simulink model "pmc_gpio_s32k11x"  (Simulink 9.0)
settings: Solver=FixedStepDiscrete  StartTime=0.0  StopTime=10.0  FixedStep=0.25  RelTol=1e-3
InitFcn:
  | mbd_s32k_consistency_checks(bdroot(gcs));
undefined symbols (not defined in the file): LQFP, thumb
libraries: mbd_s32k1xx_ec_toolbox x27, simulink x1
Description:
  | This model demonstrates the "Power Management" functionality by setting
  | the S32k144 controller in all power modes one at a time.
  | 
  | Validation: When the processor boots up, it enters the RUN power mode.  The SW3 switch
  | increments the sleep_state variable. It switches the power mode state according to the
  | sleep_state value. For every power mode, the RGB led lights up another colour:
  | RUN     - green
  | HSRUN - blue
  | STOP1 - yellow
  | STOP2 - magenta
  | VLPS   - red
  | To wake up the processor SW2 must be pressed.
  | 
  | Optional: In order to measure the current consumption of the processor you can desolder
  | the R117 resistor (on the S32K144EVB board) and attach an ammeter on the J15 jumper.
  | 
  | Warning: Do NOT program the board while the uC is running in the VLPR mode!
settings Model: Creator=NXP MBDT Team  LastModifiedBy=nxf35172
settings DataIOCC: ExternalInput=off  InitialState=off  SaveFormat=Dataset  SaveOutput=off  SignalLogging=off  SaveTime=off
settings OptimizationCC: DefaultParameterBehavior=Inlined  PassReuseOutputArgsAs=Individual arguments  LifeSpan=auto
settings DebuggingCC: UnderspecifiedInitializationDetection=Simplified  MergeDetectMultiDrivingBlocksExec=error  InheritedTsInSrcMsg=none  SingleTaskRateTransMsg=error  ParameterTunabilityLossMsg=error  UnconnectedInputMsg=error  UnconnectedOutputMsg=error  UnconnectedLineMsg=error  UnknownTsInhSupMsg=error  SFUnexpectedBacktrackingDiag=error  SFNoUnconditionalDefaultTransitionDiag=error
settings HardwareCC: ProdLargestAtomicInteger=Long  ProdLargestAtomicFloat=Double  ProdIntDivRoundTo=Zero  ProdEndianess=LittleEndian  ProdHWDeviceType=ARM Compatible->ARM Cortex
settings ModelReferenceCC: PropagateSignalLabelsOutOfModel=on
settings SFSimCC: MATLABDynamicMemAlloc=off
settings RTWCC: SystemTargetFile=mbd_s32k.tlc  MakeCommand=mbd_s32k_make_rtw COPY_MDLREF_INCLUDES=0  TemplateMakefile=mbd_s32k.tmf  Description=Model Based Design Toolbox S32K14x Code Generation Target  GenerateReport=on  RetainRTWFile=on  IncludeHyperlinkInReport=on  LaunchReport=on  GenerateTraceInfo=on  GenerateTraceReport=on  GenerateTraceReportSl=on  GenerateTraceReportSf=on  GenerateTraceReportEml=on
settings CodeAppCC: ForceParamTrailComments=on  IgnoreCustomStorageClasses=off  OperatorAnnotations=on  SimulinkDataObjDesc=on  SFDataObjDesc=on  InsertBlockDesc=on  StateflowObjectComments=off
settings STFCustomTargetCC: MultiwordLength=256  CombineOutputUpdateFcns=on  ERTCustomFileBanners=on  SupportContinuousTime=off  SupportNonInlinedSFcns=off  RemoveResetFunc=on  MATLABClassNameForMDSCustomization=Simulink.SoftwareTarget.ERTCustomization  GRTInterface=off  SystemTargetFile=mbd_s32k.tlc
settings ERTTargetCC: ParMdlRefBuildCompliant=off  CompOptLevelCompliant=off  ConcurrentExecutionCompliant=off  ModelStepFunctionPrototypeControlCompliant=off  CPPClassGenCompliant=off  UseToolchainInfoCompliant=off  InlinedParameterPlacement=NonHierarchical  ERTSrcFileBannerTemplate=mbd_ert_code_template.cgt  ERTHdrFileBannerTemplate=mbd_ert_code_template.cgt  ERTDataSrcFileTemplate=mbd_ert_code_template.cgt  ERTDataHdrFileTemplate=mbd_ert_code_template.cgt  ERTCustomFileTemplate=example_file_process.tlc
settings ConfigComp: CovMetricSettings=dwe  CovHtmlReporting=off  CovSaveCumulativeToWorkspaceVar=off  CovSaveSingleToWorkspaceVar=off  CovExternalEMLEnable=on

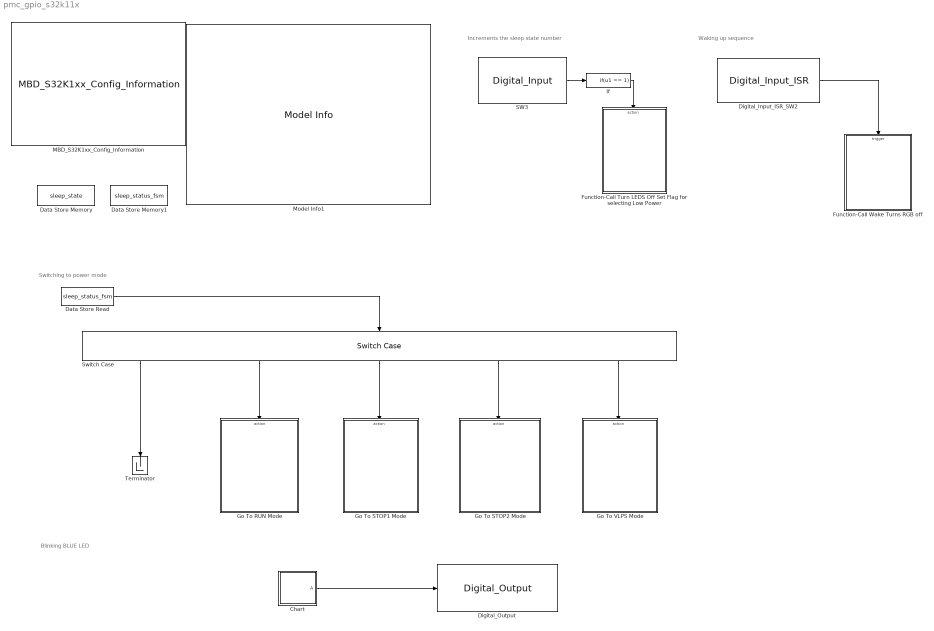
== system pmc_gpio_s32k11x ==
  note: Increments the sleep state number
  note: Waking up sequence
  note: Switching to power mode
  note: Blinking BLUE LED
  Chart : Stateflow chart  TreatAsAtomicUnit=on
  Data Store Memory : DataStoreMemory  DataStoreName=sleep_state  ReadBeforeWriteMsg=warning  WriteAfterWriteMsg=warning  WriteAfterReadMsg=warning  InitialValue=1  ShowAdditionalParam=off  OutDataTypeStr=uint8
  Data Store Memory1 : DataStoreMemory  DataStoreName=sleep_status_fsm  ReadBeforeWriteMsg=warning  WriteAfterWriteMsg=warning  WriteAfterReadMsg=warning  InitialValue=1  ShowAdditionalParam=off  OutDataTypeStr=uint8
  Data Store Read : DataStoreRead  DataStoreName=sleep_status_fsm
  Digital_Input_ISR_SW2 : mbd_s32k1xx_ec_toolbox/GPIO Blocks/Digital_Input_ISR  gpio_pin=PTD5: [PTD5 | Port D I/O]  irqc=on rising-edge  prio=0
  Digital_Output : mbd_s32k1xx_ec_toolbox/GPIO Blocks/Digital_Output  gpio_pin=PTE8: [PTE8 | Port E I/O]  init_val=Low  drive_strength=Low
  Function-Call Turn LEDS Off Set Flag for selecting Low Power : Subsystem  TreatAsAtomicUnit=on
  Function-Call Wake Turns RGB off : Subsystem  TreatAsAtomicUnit=on
  Go To RUN Mode : Subsystem  TreatAsAtomicUnit=on
  Go To STOP1 Mode : Subsystem  TreatAsAtomicUnit=on
  Go To STOP2 Mode : Subsystem  TreatAsAtomicUnit=on
  Go To VLPS Mode : Subsystem  TreatAsAtomicUnit=on
  If : If  IfExpression=u1 == 1  ShowElse=off
  MBD_S32K1xx_Config_Information : mbd_s32k1xx_ec_toolbox/MBD_S32K1xx_Config_Information  mbdt_ver=0  disp_str=|  config_params=[]  mcu_target_name=S32K116  mcu_target_package=48-LQFP  mcu_target_sram_size=17KB  mcu_system_clock_freq=40  mcu_xtal_freq=External 40  mcu_steptick_timer=LPIT Channel 0  mcu_steptick_prio=3  ds_import_enable=on  target_compiler=GCC  target_memory=FLASH  gcc_target_compile_opts=-mcpu=cortex-m0plus -mthumb -O1 -g -gstrict-dwarf  gcc_target_assemble_opts=-mcpu=cortex-m0plus -mthumb -g  gcc_target_link_opts=-mcpu=cortex-m0plus -mthumb  gcc_target_default_lcf=on  gcc_target_user_lcf=S32K116_17_flash.ld  ghs_target_compile_opts=-mcpu=cortexm0plus -mthumb -fsoft -Ogeneral -Wundef -Wimplicit-int -Wshadow -Wtrigraphs --no_commons --gnu_asm -gnu99 -gdwarf-2 -G  ghs_target_assemble_opts=-mcpu=cortexm0plus -mthumb -fsoft --gnu_asm  ghs_target_link_opts=-mcpu=cortexm0plus -mthumb -fsoft  ghs_target_default_lcf=on  ghs_target_user_lcf=S32K116_17_flash.ld  iar_target_compile_opts=--thumb -Ol -e --debug --dlib_config normal  iar_target_assemble_opts=--thumb  iar_target_link_opts=--no_exceptions --vfe --inline  iar_target_default_lcf=on  iar_target_user_lcf=S32K116_17_flash.icf  pil_download_enable=off  rbl_download_enable=on  rbl_start_delay=5000  rbl_download_interface=OpenSDA  rbl_restart_request=off  rbl_com_port=Custom  rbl_com_port_custom=COM1  pil_download_rate=57600  pil_opensda_drive=Custom  pil_opensda_drive_custom=D  pil_uart_instance=0  pil_uart_rx=PTB0: [LPUART0_RX | Receive]  pil_uart_tx=PTB1: [LPUART0_TX | Transmit]  FTM_PWM_PcrCheckEnDis=on  FTM_Input_Edge_Inputs_PcrCheckEnDis=on  FTM_Dual_Edge_Inputs_PcrCheckEnDis=on  FTM_Quadrature_Inputs_PcrCheckEnDis=on  FTM_Hall_Sensor_Inputs_PcrCheckEnDis=on  LPTMR_PcrCheckEnDis=on  PIT_PcrCheckEnDis=on  RTC_PcrCheckEnDis=on  FlexCAN_PcrCheckEnDis=on  LIN_PcrCheckEnDis=on  FlexIO_PcrCheckEnDis=on  LPI2C_PcrCheckEnDis=on  LPSPI_PcrCheckEnDis=on  LPUART_PcrCheckEnDis=on  CMP_PcrCheckEnDis=on  GPIO_OutputPcrCheckEnDis=on  GPIO_InputPcrCheckEnDis=on  SBC_PcrCheckEnDis=on  AMMCLIB_PcrCheckEnDis=on  FM_PcrCheckEnDis=on  Profile_PcrCheckEnDis=on  ConfigParams_PcrCheckEnDis=on  ModelRef_PcrCheckEnDis=on  PDB0_PcrCheckEnDis=on  CSEc_PcrCheckEnDis=on  eDMA_PcrCheckEnDis=on  ADC_PcrCheckEnDis=on  WDOG_PcrCheckEnDis=on
      | Target : S32K144-64KB_SRAM
      | Package : 100-pin
      | System clock : 80 MHz
      | XTAL clock : External 8 MHz
      | Compiler : IAR
      | Target Type : FLASH
      | Download Code after build : off
      | Step Tick Interrupt Priority : 15
  Model Info1 : simulink/Model-Wide Utilities/Model Info  Frame=off  DisplayStringWithTags=|  HorizontalTextAlignment=Left  LeftAlignmentValue=0.02
      | Model Name: %<ModelName>
      | 
      | Description: %<Description>
  SW3 : mbd_s32k1xx_ec_toolbox/GPIO Blocks/Digital_Input  gpio_pin=PTD3: [PTD3 | Port D I/O]  pull_resistor=None  passive_filter=on
  Switch Case : SwitchCase  CaseConditions={0,1,2,3,4}  ShowDefaultCase=off
  Terminator : Terminator
  wires:
  SW3/1 -> If/1
  Switch Case/1 -> Terminator/1
  Switch Case/2 -> Go To RUN Mode/Action
  If/1 -> Function-Call Turn LEDS Off Set Flag for selecting Low Power/Action
  Digital_Input_ISR_SW2/1 -> Function-Call Wake Turns RGB off/Trigger
  Data Store Read/1 -> Switch Case/1
  Chart/1(" A") -> Digital_Output/1
  Switch Case/3 -> Go To STOP1 Mode/Action
  Switch Case/4 -> Go To STOP2 Mode/Action
  Switch Case/5 -> Go To VLPS Mode/Action

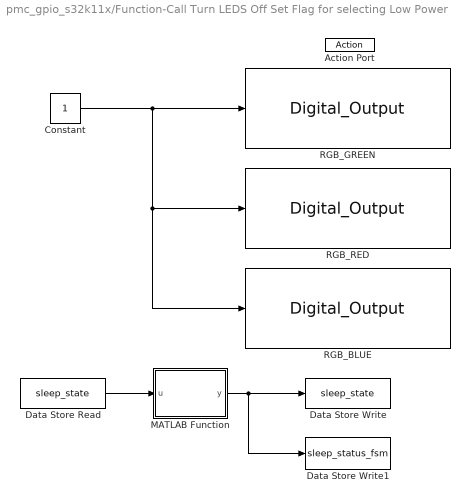
== system pmc_gpio_s32k11x/Function-Call Turn LEDS Off Set Flag for selecting Low Power ==
  Action Port : ActionPort
  Constant : Constant  OutDataTypeStr=boolean
  Data Store Read : DataStoreRead  DataStoreName=sleep_state
  Data Store Write : DataStoreWrite  DataStoreName=sleep_state
  Data Store Write1 : DataStoreWrite  DataStoreName=sleep_status_fsm
  MATLAB Function : MATLAB Function  TreatAsAtomicUnit=on
  RGB_BLUE : mbd_s32k1xx_ec_toolbox/GPIO Blocks/Digital_Output  gpio_pin=PTD0: [PTD0 | Port D I/O]  init_val=Low  drive_strength=Low
  RGB_GREEN : mbd_s32k1xx_ec_toolbox/GPIO Blocks/Digital_Output  gpio_pin=PTD16: [PTD16 | Port D I/O]  init_val=Low  drive_strength=Low
  "RGB_RED " : mbd_s32k1xx_ec_toolbox/GPIO Blocks/Digital_Output  gpio_pin=PTD15: [PTD15 | Port D I/O]  init_val=Low  drive_strength=Low
  wires:
  Constant/1 -> RGB_GREEN/1, RGB_BLUE/1, "RGB_RED "/1
  Data Store Read/1 -> MATLAB Function/1(u)
  MATLAB Function/1(y) -> Data Store Write/1, Data Store Write1/1

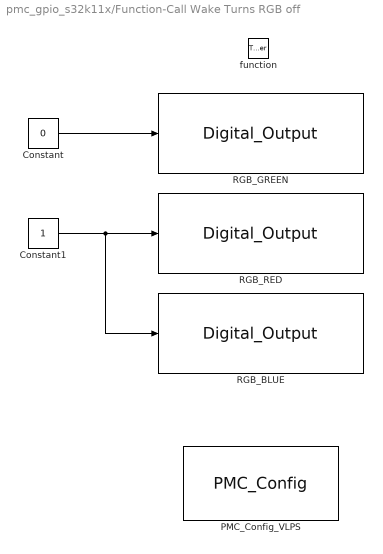
== system pmc_gpio_s32k11x/Function-Call Wake Turns RGB off ==
  function : TriggerPort  TriggerType=function-call  VariantControl=Variant
  Constant : Constant  Value=0  OutDataTypeStr=boolean
  Constant1 : Constant  OutDataTypeStr=boolean
  PMC_Config_VLPS : mbd_s32k1xx_ec_toolbox/Core and System Blocks/PMC Blocks/PMC_Config  power_mode=Normal Operating (RUN)  sleep_on_exit=off  callback_before=off  callback_after=off  callback_before_after=off  show_adv_opts=off
  RGB_BLUE : mbd_s32k1xx_ec_toolbox/GPIO Blocks/Digital_Output  gpio_pin=PTD0: [PTD0 | Port D I/O]  init_val=Low  drive_strength=Low
  RGB_GREEN : mbd_s32k1xx_ec_toolbox/GPIO Blocks/Digital_Output  gpio_pin=PTD16: [PTD16 | Port D I/O]  init_val=Low  drive_strength=Low
  "RGB_RED " : mbd_s32k1xx_ec_toolbox/GPIO Blocks/Digital_Output  gpio_pin=PTD15: [PTD15 | Port D I/O]  init_val=Low  drive_strength=Low
  wires:
  Constant/1 -> RGB_GREEN/1
  Constant1/1 -> RGB_BLUE/1, "RGB_RED "/1

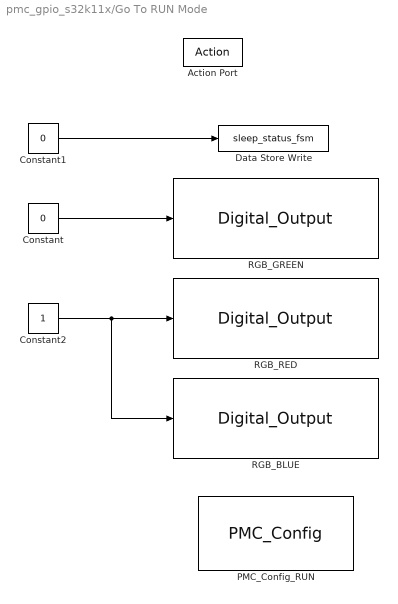
== system pmc_gpio_s32k11x/Go To RUN Mode ==
  Action Port : ActionPort
  Constant : Constant  Value=0  OutDataTypeStr=boolean
  Constant1 : Constant  Value=0  OutDataTypeStr=uint8
  Constant2 : Constant  OutDataTypeStr=boolean
  Data Store Write : DataStoreWrite  DataStoreName=sleep_status_fsm
  PMC_Config_RUN : mbd_s32k1xx_ec_toolbox/Core and System Blocks/PMC Blocks/PMC_Config  power_mode=Normal Operating (RUN)  sleep_on_exit=off  callback_before=off  callback_after=off  callback_before_after=off  show_adv_opts=off
  RGB_BLUE : mbd_s32k1xx_ec_toolbox/GPIO Blocks/Digital_Output  gpio_pin=PTE8: [PTE8 | Port E I/O]  init_val=Low  drive_strength=Low
  RGB_GREEN : mbd_s32k1xx_ec_toolbox/GPIO Blocks/Digital_Output  gpio_pin=PTD16: [PTD16 | Port D I/O]  init_val=Low  drive_strength=Low
  "RGB_RED " : mbd_s32k1xx_ec_toolbox/GPIO Blocks/Digital_Output  gpio_pin=PTD15: [PTD15 | Port D I/O]  init_val=Low  drive_strength=Low
  wires:
  Constant1/1 -> Data Store Write/1
  Constant/1 -> RGB_GREEN/1
  Constant2/1 -> RGB_BLUE/1, "RGB_RED "/1

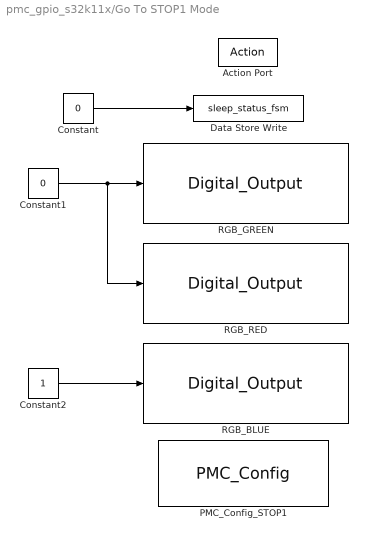
== system pmc_gpio_s32k11x/Go To STOP1 Mode ==
  Action Port : ActionPort
  Constant : Constant  Value=0  OutDataTypeStr=uint8
  Constant1 : Constant  Value=0  OutDataTypeStr=boolean
  Constant2 : Constant  OutDataTypeStr=boolean
  Data Store Write : DataStoreWrite  DataStoreName=sleep_status_fsm
  PMC_Config_STOP1 : mbd_s32k1xx_ec_toolbox/Core and System Blocks/PMC Blocks/PMC_Config  power_mode=Stop System and Bus clocks (STOP1)  sleep_on_exit=off  callback_before=off  callback_after=off  callback_before_after=off  show_adv_opts=on
  RGB_BLUE : mbd_s32k1xx_ec_toolbox/GPIO Blocks/Digital_Output  gpio_pin=PTE8: [PTE8 | Port E I/O]  init_val=Low  drive_strength=Low
  RGB_GREEN : mbd_s32k1xx_ec_toolbox/GPIO Blocks/Digital_Output  gpio_pin=PTD16: [PTD16 | Port D I/O]  init_val=Low  drive_strength=Low
  "RGB_RED " : mbd_s32k1xx_ec_toolbox/GPIO Blocks/Digital_Output  gpio_pin=PTD15: [PTD15 | Port D I/O]  init_val=Low  drive_strength=Low
  wires:
  Constant2/1 -> RGB_BLUE/1
  Constant1/1 -> RGB_GREEN/1, "RGB_RED "/1
  Constant/1 -> Data Store Write/1

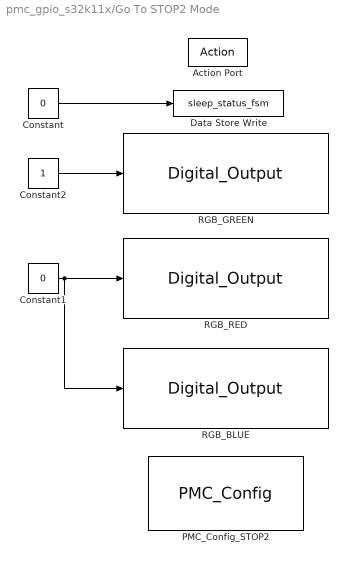
== system pmc_gpio_s32k11x/Go To STOP2 Mode ==
  Action Port : ActionPort
  Constant : Constant  Value=0  OutDataTypeStr=uint8
  Constant1 : Constant  Value=0  OutDataTypeStr=boolean
  Constant2 : Constant  OutDataTypeStr=boolean
  Data Store Write : DataStoreWrite  DataStoreName=sleep_status_fsm
  PMC_Config_STOP2 : mbd_s32k1xx_ec_toolbox/Core and System Blocks/PMC Blocks/PMC_Config  power_mode=Stop System clock and keep Bus clock running (STOP2)  sleep_on_exit=off  callback_before=off  callback_after=off  callback_before_after=off  show_adv_opts=off
  RGB_BLUE : mbd_s32k1xx_ec_toolbox/GPIO Blocks/Digital_Output  gpio_pin=PTE8: [PTE8 | Port E I/O]  init_val=Low  drive_strength=Low
  RGB_GREEN : mbd_s32k1xx_ec_toolbox/GPIO Blocks/Digital_Output  gpio_pin=PTD16: [PTD16 | Port D I/O]  init_val=Low  drive_strength=Low
  "RGB_RED " : mbd_s32k1xx_ec_toolbox/GPIO Blocks/Digital_Output  gpio_pin=PTD15: [PTD15 | Port D I/O]  init_val=Low  drive_strength=Low
  wires:
  Constant/1 -> Data Store Write/1
  Constant1/1 -> RGB_BLUE/1, "RGB_RED "/1
  Constant2/1 -> RGB_GREEN/1

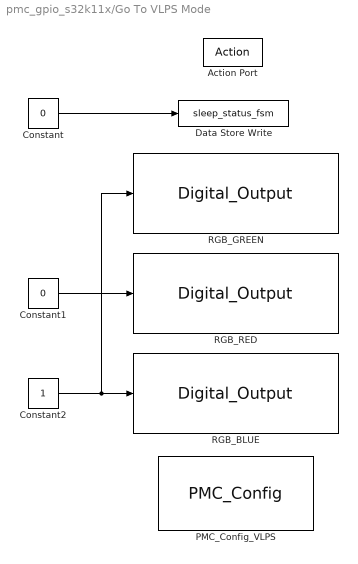
== system pmc_gpio_s32k11x/Go To VLPS Mode ==
  Action Port : ActionPort
  Constant : Constant  Value=0  OutDataTypeStr=uint8
  Constant1 : Constant  Value=0  OutDataTypeStr=boolean
  Constant2 : Constant  OutDataTypeStr=boolean
  Data Store Write : DataStoreWrite  DataStoreName=sleep_status_fsm
  PMC_Config_VLPS : mbd_s32k1xx_ec_toolbox/Core and System Blocks/PMC Blocks/PMC_Config  power_mode=Very Low Power Stop (VLPS)  sleep_on_exit=off  callback_before=off  callback_after=off  callback_before_after=off  show_adv_opts=off
  RGB_BLUE : mbd_s32k1xx_ec_toolbox/GPIO Blocks/Digital_Output  gpio_pin=PTE8: [PTE8 | Port E I/O]  init_val=Low  drive_strength=Low
  RGB_GREEN : mbd_s32k1xx_ec_toolbox/GPIO Blocks/Digital_Output  gpio_pin=PTD16: [PTD16 | Port D I/O]  init_val=Low  drive_strength=Low
  "RGB_RED " : mbd_s32k1xx_ec_toolbox/GPIO Blocks/Digital_Output  gpio_pin=PTD15: [PTD15 | Port D I/O]  init_val=Low  drive_strength=Low
  wires:
  Constant/1 -> Data Store Write/1
  Constant2/1 -> RGB_GREEN/1, RGB_BLUE/1
  Constant1/1 -> "RGB_RED "/1

== matlab function Function-Call Turn LEDS Off Set Flag for selecting Low Power/MATLAB Function ==
  data: u input double; y output double
function y = fcn(u)

y = mod(u + 1, 7);

== stateflow chart Chart ==
  state A
  state A1
  (default) -> A
  A -> A1
  A1 -> A
  data: A output boolean [0..1]
